simulink model "lab_4_4_bpsk_fixed_point_chain"  (R2025a)
settings: Solver=FixedStepDiscrete  StartTime=0.0  StopTime=lab44_fixed_chain_stop_time  FixedStep=1  RelTol=1e-3
InitFcn:
  | lab_4_4_ensure_bpsk_simulink_workspace;
undefined symbols (not defined in the file): lab44_rrc_taps_q15, lab44_tx_gain
libraries: simulink x1
settings Model: Creator=user  LastModifiedBy=user

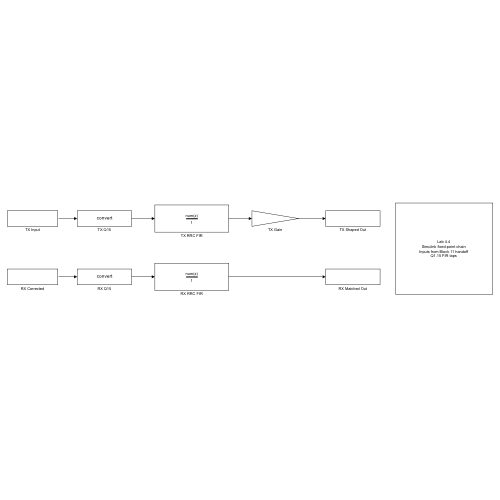
[thumbnail: Simulink's stored preview of the top-level diagram]
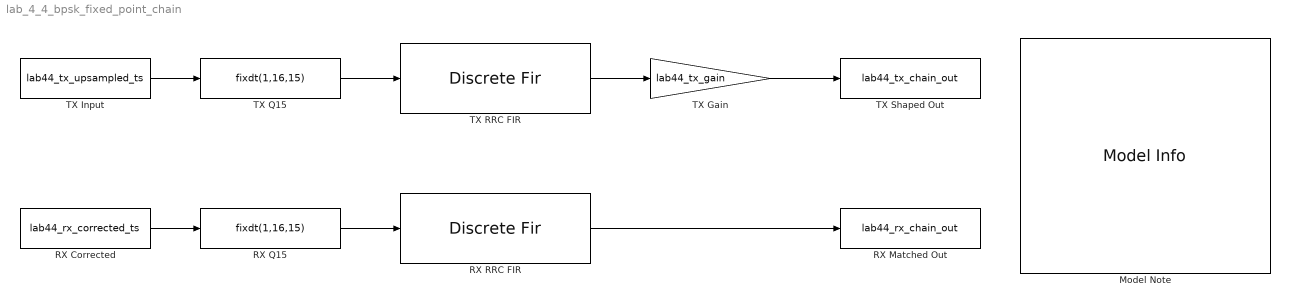
== system lab_4_4_bpsk_fixed_point_chain ==
  Model Note : simulink/Model-Wide Utilities/Model Info  Frame=on  DisplayStringWithTags=Model Info  HorizontalTextAlignment=Center  LeftAlignmentValue=0.5
  RX Corrected : FromWorkspace  VariableName=lab44_rx_corrected_ts
  RX Matched Out : ToWorkspace  VariableName=lab44_rx_chain_out  SaveFormat=Timeseries  SampleTime=-1
  RX Q15 : DataTypeConversion  OutDataTypeStr=fixdt(1,16,15)  SaturateOnIntegerOverflow=off  RndMeth=Floor
  RX RRC FIR : DiscreteFir  Coefficients=lab44_rrc_taps_q15.'  ProductDataTypeStr=fixdt(1,32,30)  AccumDataTypeStr=fixdt(1,40,30)  OutDataTypeStr=fixdt(1,40,30)  RndMeth=Nearest  SaturateOnIntegerOverflow=on
  TX Gain : Gain  Gain=lab44_tx_gain
  TX Input : FromWorkspace  VariableName=lab44_tx_upsampled_ts
  TX Q15 : DataTypeConversion  OutDataTypeStr=fixdt(1,16,15)  SaturateOnIntegerOverflow=off  RndMeth=Floor
  TX RRC FIR : DiscreteFir  Coefficients=lab44_rrc_taps_q15.'  ProductDataTypeStr=fixdt(1,32,30)  AccumDataTypeStr=fixdt(1,40,30)  OutDataTypeStr=fixdt(1,40,30)  RndMeth=Nearest  SaturateOnIntegerOverflow=on
  TX Shaped Out : ToWorkspace  VariableName=lab44_tx_chain_out  SaveFormat=Timeseries  SampleTime=-1
  wires:
  TX Input/1 -> TX Q15/1
  TX Q15/1 -> TX RRC FIR/1
  TX RRC FIR/1 -> TX Gain/1
  TX Gain/1 -> TX Shaped Out/1
  RX Corrected/1 -> RX Q15/1
  RX Q15/1 -> RX RRC FIR/1
  RX RRC FIR/1 -> RX Matched Out/1
